simulink model "hx_sim"  (R2017b)
settings: Solver=ode23tb  StartTime=0.0  StopTime=tEndSimul  MaxStep=0.1  RelTol=5e-6
values from neighbouring files (symbols this model uses):
  dnDt_in = mass_flow_converter(0.020, 'kg/min', 'mol/sec', 'Ammonia')    [hx.m]
  dnDt_out_liq = mass_flow_converter(0.020, 'kg/min', 'mol/sec', 'Ammonia')    [hx.m]
  dnDt_out_vap = mass_flow_converter(0, 'kg/h', 'mol/sec', 'Ammonia')    [hx.m]
  fluid = nh3_v4    [hx.m]
  h_inner_liq = 1e2    (= 100)    [hx.m]
  h_inner_vap = 1e4    (= 10000)    [hx.m]
  h_outer = 200    [hx.m]
  Nhx_init = Vhx/10 * rho_nh3_Tamb    [hx.m]
  T_dnDt_in_C = 120    [hx.m]
  Tamb_C = 25    [hx.m]
  tEnd_dnDt_in = tStart_dnDt_in + 10 * c.min_to_sec    [hx.m]
  tEnd_dnDt_out_liq = tStart_dnDt_out_liq + 10 * c.min_to_sec    [hx.m]
  tEnd_dnDt_out_vap = tStart_dnDt_out_vap + 0 * c.min_to_sec    [hx.m]
  Thx_init = c.C_to_K(Tamb_C)    [hx.m]
  Tout1_C = (20+30)/2    (= 25)    [hx.m]
  tStart_dnDt_in = 10 * c.min_to_sec    [hx.m]
  tStart_dnDt_out_liq = tEnd_dnDt_in + 5 * c.min_to_sec    [hx.m]
  tStart_dnDt_out_vap = 0    [hx.m]
  Vhx = 0.5 * c.L_to_m3    [hx.m]
undefined symbols (not defined in the file or in its folder): h, P, T
libraries: thermochemical x19, simulink x4
settings Model: Creator=ferru  LastModifiedBy=fferrucc
settings SolverCC: AlgebraicLoopSolver=LineSearch

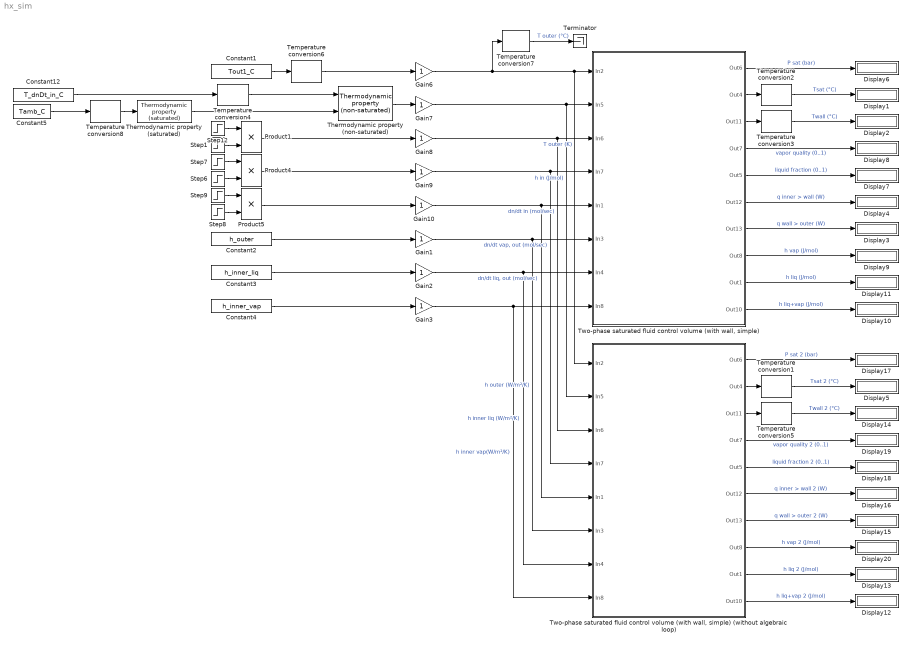
== system hx_sim ==
  Constant1 : Constant  Value=Tout1_C
  Constant12 : Constant  Value=T_dnDt_in_C
  Constant2 : Constant  Value=h_outer
  Constant3 : Constant  Value=h_inner_liq
  Constant4 : Constant  Value=h_inner_vap
  Constant5 : Constant  Value=Tamb_C
  Display{1..20} (20 alike) : Display
  Gain{1..3,6..10} (8 alike) : Gain
  Product1 : Product
  Product4 : Product
  Product5 : Product
  Step1 : Step  Time=tEnd_dnDt_in  Before=1  After=0  SampleTime=0
  Step12 : Step  Time=tStart_dnDt_in  After=dnDt_in  SampleTime=0
  Step6 : Step  Time=tEnd_dnDt_out_vap  Before=1  After=0  SampleTime=0
  Step7 : Step  Time=tStart_dnDt_out_vap  After=dnDt_out_vap  SampleTime=0
  Step8 : Step  Time=tEnd_dnDt_out_liq  Before=1  After=0  SampleTime=0
  Step9 : Step  Time=tStart_dnDt_out_liq  After=dnDt_out_liq  SampleTime=0
  Temperature conversion{1..3,5,7} (5 alike) : thermochemical/Conversions/Temperature conversion  sel=K --> °C
      settings: SourceProductName=@ Thermochemical
  Temperature conversion4 : thermochemical/Conversions/Temperature conversion  sel=°C --> K
      settings: SourceProductName=@ Thermochemical
  Temperature conversion6 : thermochemical/Conversions/Temperature conversion  sel=°C --> K
      settings: SourceProductName=@ Thermochemical
  Temperature conversion8 : thermochemical/Conversions/Temperature conversion  sel=°C --> K
      settings: SourceProductName=@ Thermochemical
  Terminator : Terminator
  Thermodynamic property (non-saturated) : thermochemical/Thermodynamic fluid properties/Thermodynamic  property (non-saturated)  sel=h(T,P)  fluid=fluid  reciprocVar=-1  lookup2D_BreakPoint1=fluid.no_sat.T_P_indep.var_indep.T  lookup2D_BreakPoint2=fluid.no_sat.T_P_indep.var_indep.P  lookup2D_Data=fluid.no_sat.T_P_indep.var_dep.h_molar
      settings: SourceProductName=@ Thermochemical
  Thermodynamic property (saturated) : thermochemical/Thermodynamic fluid properties/Thermodynamic  property (saturated)  sel=P(T) (bar)  fluid=fluid  lookup1D_BreakPoint1=fluid.sat.T  lookup1D_Data=fluid.sat.Psat
      settings: SourceProductName=@ Thermochemical
  "Two-phase saturated fluid control volume (with wall, simple)" : Subsystem  AncestorBlock=|
      | thermochemical/Control volumes/Two-phase saturated fluid
      | control volume (with wall, simple)
  "Two-phase saturated fluid control volume (with wall, simple) (without algebraic loop)" : Subsystem  AncestorBlock=|
      | thermochemical/Control volumes/Two-phase saturated fluid
      | control volume (with wall, simple)
      | (without algebraic loop)
  wires:
  Step12/1 -> Product1/1
  Step1/1 -> Product1/2
  Constant12/1 -> Temperature conversion4/1
  Temperature conversion4/1 -> Thermodynamic property (non-saturated)/1
  Temperature conversion2/1 -> Display1/1  "Tsat (°C)"
  "Two-phase saturated fluid control volume (with wall, simple)"/2(Out4) -> Temperature conversion2/1
  Gain6/1 -> Temperature conversion7/1, "Two-phase saturated fluid control volume (with wall, simple) (without algebraic loop)"/1(In2), "Two-phase saturated fluid control volume (with wall, simple)"/1(In2)  "T outer (K)"
  Gain7/1 -> "Two-phase saturated fluid control volume (with wall, simple) (without algebraic loop)"/2(In5), "Two-phase saturated fluid control volume (with wall, simple)"/2(In5)  "h in (J/mol)"
  Gain8/1 -> "Two-phase saturated fluid control volume (with wall, simple) (without algebraic loop)"/3(In6), "Two-phase saturated fluid control volume (with wall, simple)"/3(In6)  "dn/dt in (mol/sec)"
  Gain9/1 -> "Two-phase saturated fluid control volume (with wall, simple) (without algebraic loop)"/4(In7), "Two-phase saturated fluid control volume (with wall, simple)"/4(In7)  "dn/dt vap, out (mol/sec)"
  Gain10/1 -> "Two-phase saturated fluid control volume (with wall, simple) (without algebraic loop)"/5(In1), "Two-phase saturated fluid control volume (with wall, simple)"/5(In1)  "dn/dt liq, out (mol/sec)"
  "Two-phase saturated fluid control volume (with wall, simple)"/1(Out6) -> Display6/1  "P sat (bar)"
  "Two-phase saturated fluid control volume (with wall, simple)"/5(Out5) -> Display7/1  "liquid fraction (0..1)"
  "Two-phase saturated fluid control volume (with wall, simple)"/4(Out7) -> Display8/1  "vapor quality (0..1)"
  "Two-phase saturated fluid control volume (with wall, simple)"/8(Out8) -> Display9/1  "h vap (J/mol)"
  "Two-phase saturated fluid control volume (with wall, simple)"/10(Out10) -> Display10/1  "h liq+vap (J/mol)"
  "Two-phase saturated fluid control volume (with wall, simple)"/9(Out1) -> Display11/1  "h liq (J/mol)"
  Constant1/1 -> Temperature conversion6/1
  Thermodynamic property (non-saturated)/1 -> Gain7/1
  Product1/1 -> Gain8/1
  Product4/1 -> Gain9/1
  Step6/1 -> Product4/2
  Step7/1 -> Product4/1
  Step9/1 -> Product5/1
  Step8/1 -> Product5/2
  Product5/1 -> Gain10/1
  "Two-phase saturated fluid control volume (with wall, simple)"/3(Out11) -> Temperature conversion3/1
  Temperature conversion3/1 -> Display2/1  "Twall (°C)"
  "Two-phase saturated fluid control volume (with wall, simple)"/7(Out13) -> Display3/1  "q wall > outer (W)"
  "Two-phase saturated fluid control volume (with wall, simple)"/6(Out12) -> Display4/1  "q inner > wall (W)"
  "Two-phase saturated fluid control volume (with wall, simple) (without algebraic loop)"/6(Out12) -> Display16/1  "q inner > wall 2 (W)"
  "Two-phase saturated fluid control volume (with wall, simple) (without algebraic loop)"/7(Out13) -> Display15/1  "q wall > outer 2 (W)"
  Temperature conversion5/1 -> Display14/1  "Twall 2 (°C)"
  "Two-phase saturated fluid control volume (with wall, simple) (without algebraic loop)"/3(Out11) -> Temperature conversion5/1
  "Two-phase saturated fluid control volume (with wall, simple) (without algebraic loop)"/9(Out1) -> Display13/1  "h liq 2 (J/mol)"
  "Two-phase saturated fluid control volume (with wall, simple) (without algebraic loop)"/10(Out10) -> Display12/1  "h liq+vap 2 (J/mol)"
  "Two-phase saturated fluid control volume (with wall, simple) (without algebraic loop)"/8(Out8) -> Display20/1  "h vap 2 (J/mol)"
  "Two-phase saturated fluid control volume (with wall, simple) (without algebraic loop)"/4(Out7) -> Display19/1  "vapor quality 2 (0..1)"
  "Two-phase saturated fluid control volume (with wall, simple) (without algebraic loop)"/5(Out5) -> Display18/1  "liquid fraction 2 (0..1)"
  "Two-phase saturated fluid control volume (with wall, simple) (without algebraic loop)"/1(Out6) -> Display17/1  "P sat 2 (bar)"
  "Two-phase saturated fluid control volume (with wall, simple) (without algebraic loop)"/2(Out4) -> Temperature conversion1/1
  Temperature conversion1/1 -> Display5/1  "Tsat 2 (°C)"
  Temperature conversion6/1 -> Gain6/1
  Temperature conversion7/1 -> Terminator/1  "T outer (°C)"
  Gain3/1 -> "Two-phase saturated fluid control volume (with wall, simple) (without algebraic loop)"/8(In8), "Two-phase saturated fluid control volume (with wall, simple)"/8(In8)  "h inner vap(W/m²/K)"
  Gain1/1 -> "Two-phase saturated fluid control volume (with wall, simple)"/6(In3), "Two-phase saturated fluid control volume (with wall, simple) (without algebraic loop)"/6(In3)  "h outer (W/m²/K)"
  Gain2/1 -> "Two-phase saturated fluid control volume (with wall, simple) (without algebraic loop)"/7(In4), "Two-phase saturated fluid control volume (with wall, simple)"/7(In4)  "h inner liq (W/m²/K)"
  Constant2/1 -> Gain1/1
  Constant3/1 -> Gain2/1
  Constant4/1 -> Gain3/1
  Constant5/1 -> Temperature conversion8/1
  Temperature conversion8/1 -> Thermodynamic property (saturated)/1
  Thermodynamic property (saturated)/1 -> Thermodynamic property (non-saturated)/2

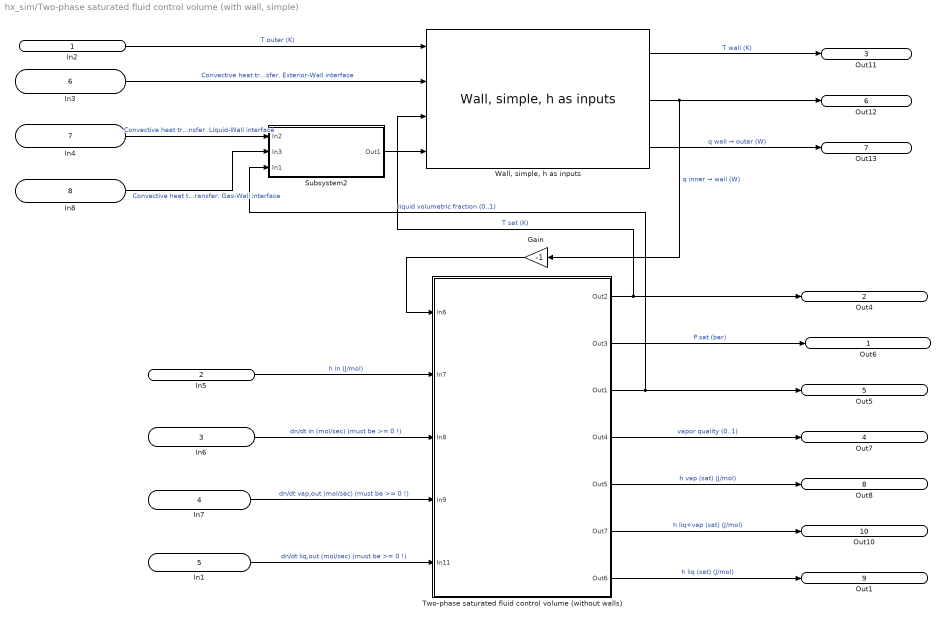
== system hx_sim/Two-phase saturated fluid control volume (with wall, simple) ==
  In2 : Inport
  In5 : Inport  Port=2
  In6 : Inport  Port=3
  In7 : Inport  Port=4
  In1 : Inport  Port=5
  In3 : Inport  Port=6
  In4 : Inport  Port=7
  In8 : Inport  Port=8
  Gain : Gain  Gain=-1
  Subsystem2 : Subsystem
  Two-phase saturated fluid control volume (without walls) : Subsystem  AncestorBlock=|  mask(volume_control_saturated){N_init=Nhx_init, T_init=Thx_init, fluid=fluid, V=Vhx}
      | thermochemical/Control volumes/Two-phase saturated fluid
      | control volume (without walls)
      mask prompts: N_init "Initial number of mols inside the control volume (mol)"; T_init "Fluid initial temperature (K)"; fluid "Fluid (structure data type)"; V "Volume (m3)"
      mask help:
      | This block models a volume control that contains a fluid always in its saturation state.
      |
      | The model can work as a condenser or as an evaporator:
      | • Condenser: connect the output 'h liq (J/mol)' to the input 'h out (sat) (J/mol)'
      | • Evaporator: connect the output 'h vap (J/mol)' to the input 'h out (sat) (J/mol)'
      |
      | The ratio between the two phases is given by two outputs:
      | 1) volumetric liquid fraction: liquid volume/total volume (0..1)
      | 2) vapor quality (e.g. zero: 100% liquid, one: 100% vapor).
      |
      | Note 2: the model is not prepared to work in the non-saturation state of the fluid (e.g. superheated gas or supercooled liquid). This means that both the liquid fraction and the vapor quality are strictly constrained in the (0..1) open range. The simulation will stop if these constrains are violated.
      mask DialogControl Container3 Prompt: Initial state
      mask DialogControl Container4 Prompt: Other parameters
  "Wall, simple, h as inputs" : thermochemical/Walls/Wall, simple, h as inputs  material=Stainless steel AISI316  cp=490.8  rho=8023  s=Shx_m2  e_mm=thickness_hx_mm  mass=2.2529  Twall_init=Thx_init
      settings: SourceProductName=@ Thermochemical
  Out6 : Outport
  Out4 : Outport  Port=2
  Out11 : Outport  Port=3
  Out7 : Outport  Port=4
  Out5 : Outport  Port=5
  Out12 : Outport  Port=6
  Out13 : Outport  Port=7
  Out8 : Outport  Port=8
  Out1 : Outport  Port=9
  Out10 : Outport  Port=10
  wires:
  Subsystem2/1(Out1) -> "Wall, simple, h as inputs"/4
  "Wall, simple, h as inputs"/2 -> Gain/1, Out12/1  "q inner → wall (W)"
  "Wall, simple, h as inputs"/1 -> Out11/1  "T wall (K)"
  In3/1 -> "Wall, simple, h as inputs"/2  "Convective heat transfer. Exterior-Wall interface"
  In4/1 -> Subsystem2/1(In2)  "Convective heat transfer. Liquid-Wall interface"
  Two-phase saturated fluid control volume (without walls)/7(Out6) -> Out1/1  "h liq (sat) (J/mol)"
  Two-phase saturated fluid control volume (without walls)/1(Out2) -> "Wall, simple, h as inputs"/3, Out4/1  "T sat (K)"
  Two-phase saturated fluid control volume (without walls)/2(Out3) -> Out6/1  "P sat (bar)"
  Two-phase saturated fluid control volume (without walls)/6(Out7) -> Out10/1  "h liq+vap (sat) (J/mol)"
  In7/1 -> Two-phase saturated fluid control volume (without walls)/4(In9)  "dn/dt vap,out (mol/sec) (must be >= 0 !)"
  Two-phase saturated fluid control volume (without walls)/5(Out5) -> Out8/1  "h vap (sat) (J/mol)"
  Two-phase saturated fluid control volume (without walls)/4(Out4) -> Out7/1  "vapor quality (0..1)"
  Two-phase saturated fluid control volume (without walls)/3(Out1) -> Subsystem2/3(In1), Out5/1  "liquid volumetric fraction (0..1)"
  In5/1 -> Two-phase saturated fluid control volume (without walls)/2(In7)  "h in (J/mol)"
  In6/1 -> Two-phase saturated fluid control volume (without walls)/3(In8)  "dn/dt in (mol/sec) (must be >= 0 !)"
  In8/1 -> Subsystem2/2(In3)  "Convective heat transfer. Gas-Wall interface"
  "Wall, simple, h as inputs"/3 -> Out13/1  "q wall → outer (W)"
  In2/1 -> "Wall, simple, h as inputs"/1  "T outer (K)"
  Gain/1 -> Two-phase saturated fluid control volume (without walls)/1(In6)
  In1/1 -> Two-phase saturated fluid control volume (without walls)/5(In11)  "dn/dt liq,out (mol/sec) (must be >= 0 !)"

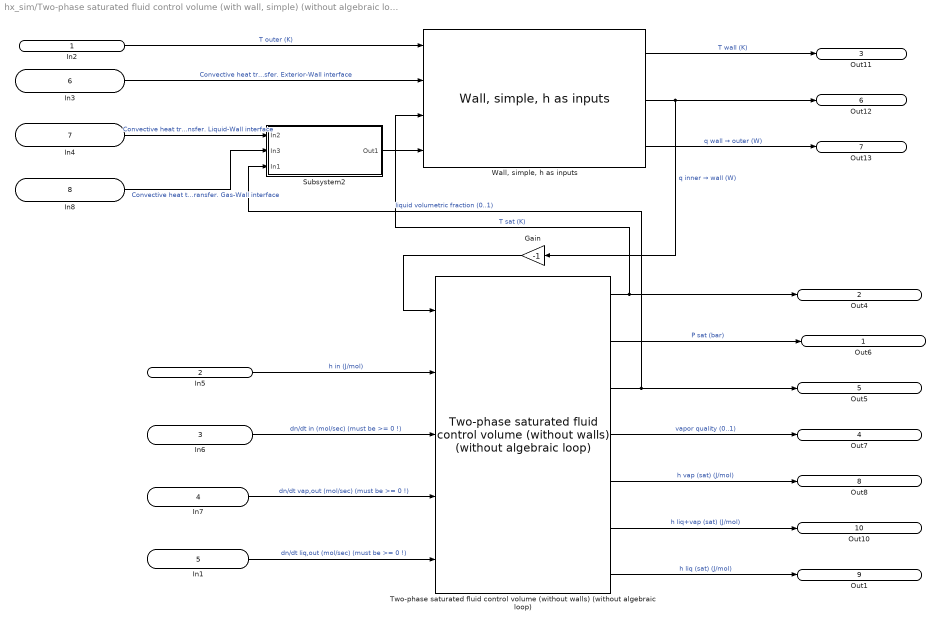
== system hx_sim/Two-phase saturated fluid control volume (with wall, simple) (without algebraic loop) ==
  In2 : Inport
  In5 : Inport  Port=2
  In6 : Inport  Port=3
  In7 : Inport  Port=4
  In1 : Inport  Port=5
  In3 : Inport  Port=6
  In4 : Inport  Port=7
  In8 : Inport  Port=8
  Gain : Gain  Gain=-1
  Subsystem2 : Subsystem
  Two-phase saturated fluid control volume (without walls) (without algebraic loop) : thermochemical/Control volumes/Two-phase saturated fluid control volume (without walls) (without algebraic loop)  N_init=Nhx_init  T_init=Thx_init  fluid=fluid  V=Vhx
      settings: SourceProductName=@ Thermochemical
  "Wall, simple, h as inputs" : thermochemical/Walls/Wall, simple, h as inputs  material=Stainless steel AISI316  cp=490.8  rho=8023  s=Shx_m2  e_mm=thickness_hx_mm  mass=2.2529  Twall_init=Thx_init
      settings: SourceProductName=@ Thermochemical
  Out6 : Outport
  Out4 : Outport  Port=2
  Out11 : Outport  Port=3
  Out7 : Outport  Port=4
  Out5 : Outport  Port=5
  Out12 : Outport  Port=6
  Out13 : Outport  Port=7
  Out8 : Outport  Port=8
  Out1 : Outport  Port=9
  Out10 : Outport  Port=10
  wires:
  In1/1 -> Two-phase saturated fluid control volume (without walls) (without algebraic loop)/5  "dn/dt liq,out (mol/sec) (must be >= 0 !)"
  Gain/1 -> Two-phase saturated fluid control volume (without walls) (without algebraic loop)/1
  In2/1 -> "Wall, simple, h as inputs"/1  "T outer (K)"
  "Wall, simple, h as inputs"/3 -> Out13/1  "q wall → outer (W)"
  In6/1 -> Two-phase saturated fluid control volume (without walls) (without algebraic loop)/3  "dn/dt in (mol/sec) (must be >= 0 !)"
  In5/1 -> Two-phase saturated fluid control volume (without walls) (without algebraic loop)/2  "h in (J/mol)"
  Two-phase saturated fluid control volume (without walls) (without algebraic loop)/3 -> Out5/1, Subsystem2/3(In1)  "liquid volumetric fraction (0..1)"
  Two-phase saturated fluid control volume (without walls) (without algebraic loop)/4 -> Out7/1  "vapor quality (0..1)"
  Two-phase saturated fluid control volume (without walls) (without algebraic loop)/5 -> Out8/1  "h vap (sat) (J/mol)"
  In7/1 -> Two-phase saturated fluid control volume (without walls) (without algebraic loop)/4  "dn/dt vap,out (mol/sec) (must be >= 0 !)"
  Two-phase saturated fluid control volume (without walls) (without algebraic loop)/6 -> Out10/1  "h liq+vap (sat) (J/mol)"
  Two-phase saturated fluid control volume (without walls) (without algebraic loop)/2 -> Out6/1  "P sat (bar)"
  Two-phase saturated fluid control volume (without walls) (without algebraic loop)/1 -> Out4/1, "Wall, simple, h as inputs"/3  "T sat (K)"
  Two-phase saturated fluid control volume (without walls) (without algebraic loop)/7 -> Out1/1  "h liq (sat) (J/mol)"
  "Wall, simple, h as inputs"/1 -> Out11/1  "T wall (K)"
  "Wall, simple, h as inputs"/2 -> Out12/1, Gain/1  "q inner → wall (W)"
  Subsystem2/1(Out1) -> "Wall, simple, h as inputs"/4
  In4/1 -> Subsystem2/1(In2)  "Convective heat transfer. Liquid-Wall interface"
  In3/1 -> "Wall, simple, h as inputs"/2  "Convective heat transfer. Exterior-Wall interface"
  In8/1 -> Subsystem2/2(In3)  "Convective heat transfer. Gas-Wall interface"

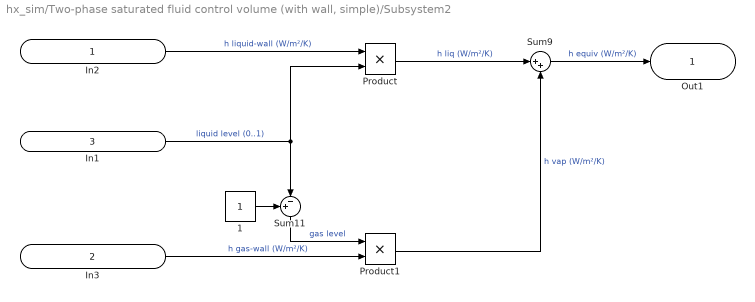
== system hx_sim/Two-phase saturated fluid control volume (with wall, simple)/Subsystem2 ==
  In2 : Inport
  In3 : Inport  Port=2
  In1 : Inport  Port=3
  1 : Constant
  Product : Product
  Product1 : Product
  Sum11 : Sum  Inputs=+-|
  Sum9 : Sum  Inputs=|++
  Out1 : Outport
  wires:
  Sum9/1 -> Out1/1  "h equiv (W/m²/K)"
  In1/1 -> Product/2, Sum11/2  "liquid level (0..1)"
  In3/1 -> Product1/2  "h gas-wall (W/m²/K)"
  In2/1 -> Product/1  "h liquid-wall (W/m²/K)"
  Sum11/1 -> Product1/1  "gas level"
  1/1 -> Sum11/1
  Product1/1 -> Sum9/2  "h vap (W/m²/K)"
  Product/1 -> Sum9/1  "h liq (W/m²/K)"

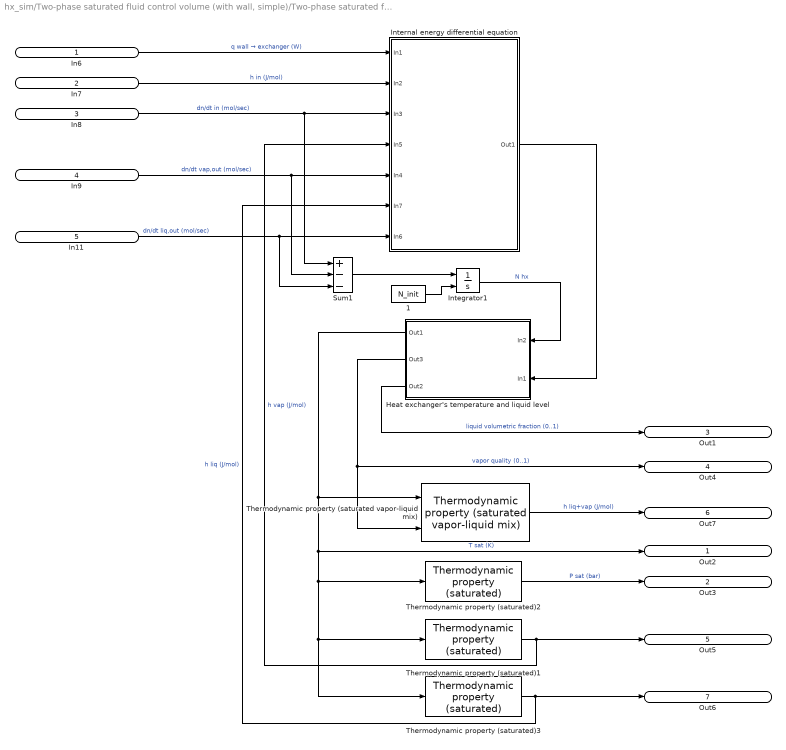
== system hx_sim/Two-phase saturated fluid control volume (with wall, simple)/Two-phase saturated fluid control volume (without walls) ==
  In6 : Inport
  In7 : Inport  Port=2
  In8 : Inport  Port=3
  In9 : Inport  Port=4
  In11 : Inport  Port=5
  1 : Constant  Value=N_init
  Heat exchanger's temperature and liquid level : Subsystem
  Integrator1 : Integrator  InitialConditionSource=external  InitialCondition=N_init
  Internal energy differential equation : Subsystem
  Sum1 : Sum  Inputs=+--
  Thermodynamic property (saturated)1 : thermochemical/Thermodynamic fluid properties/Thermodynamic  property (saturated)  sel=h(T) vap. (J/mol)  fluid=fluid  lookup1D_BreakPoint1=fluid.sat.T  lookup1D_Data=fluid.sat.vap.h_molar
      settings: SourceProductName=@ Thermochemical
  Thermodynamic property (saturated)2 : thermochemical/Thermodynamic fluid properties/Thermodynamic  property (saturated)  sel=P(T) (bar)  fluid=fluid  lookup1D_BreakPoint1=fluid.sat.T  lookup1D_Data=fluid.sat.Psat
      settings: SourceProductName=@ Thermochemical
  Thermodynamic property (saturated)3 : thermochemical/Thermodynamic fluid properties/Thermodynamic  property (saturated)  sel=h(T) liq. (J/mol)  fluid=fluid  lookup1D_BreakPoint1=fluid.sat.T  lookup1D_Data=fluid.sat.liq.h_molar
      settings: SourceProductName=@ Thermochemical
  Thermodynamic property (saturated vapor-liquid mix) : thermochemical/Thermodynamic fluid properties/Thermodynamic property  (saturated vapor-liquid mix)  sel=h(T) (J/mol)  fluid=fluid  lookup1D_BreakPoint=0  lookup1D_Data1=fluid.sat.liq.h_molar  lookup1D_Data2=fluid.sat.vap.h_molar
      settings: SourceProductName=@ Thermochemical
  Out2 : Outport
  Out3 : Outport  Port=2
  Out1 : Outport  Port=3
  Out4 : Outport  Port=4
  Out5 : Outport  Port=5
  Out7 : Outport  Port=6
  Out6 : Outport  Port=7
  wires:
  1/1 -> Integrator1/2
  In7/1 -> Internal energy differential equation/2(In2)  "h in (J/mol)"
  In11/1 -> Internal energy differential equation/7(In6), Sum1/3  "dn/dt liq,out (mol/sec)"
  In8/1 -> Internal energy differential equation/3(In3), Sum1/1  "dn/dt in (mol/sec)"
  In6/1 -> Internal energy differential equation/1(In1)  "q wall → exchanger (W)"
  In9/1 -> Internal energy differential equation/5(In4), Sum1/2  "dn/dt vap,out (mol/sec)"
  Thermodynamic property (saturated)3/1 -> Internal energy differential equation/6(In7), Out6/1  "h liq (J/mol)"
  Thermodynamic property (saturated vapor-liquid mix)/1 -> Out7/1  "h liq+vap (J/mol)"
  Thermodynamic property (saturated)1/1 -> Out5/1, Internal energy differential equation/4(In5)  "h vap (J/mol)"
  Internal energy differential equation/1(Out1) -> Heat exchanger's temperature and liquid level/2(In1)
  Integrator1/1 -> Heat exchanger's temperature and liquid level/1(In2)  "N hx"
  Heat exchanger's temperature and liquid level/2(Out3) -> Out4/1, Thermodynamic property (saturated vapor-liquid mix)/2  "vapor quality (0..1)"
  Thermodynamic property (saturated)2/1 -> Out3/1  "P sat (bar)"
  Heat exchanger's temperature and liquid level/1(Out1) -> Thermodynamic property (saturated vapor-liquid mix)/1, Out2/1, Thermodynamic property (saturated)2/1, Thermodynamic property (saturated)1/1, Thermodynamic property (saturated)3/1  "T sat (K)"
  Heat exchanger's temperature and liquid level/3(Out2) -> Out1/1  "liquid volumetric fraction (0..1)"
  Sum1/1 -> Integrator1/1

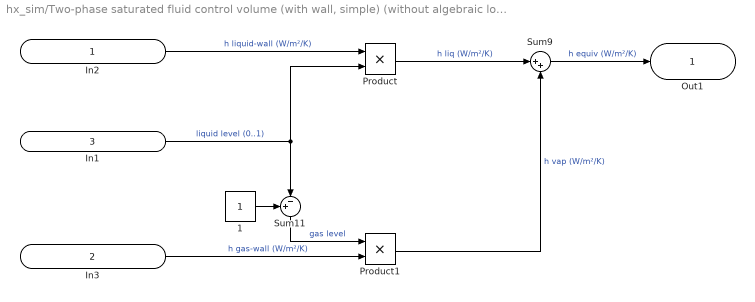
== system hx_sim/Two-phase saturated fluid control volume (with wall, simple) (without algebraic loop)/Subsystem2 ==
  In2 : Inport
  In3 : Inport  Port=2
  In1 : Inport  Port=3
  1 : Constant
  Product : Product
  Product1 : Product
  Sum11 : Sum  Inputs=+-|
  Sum9 : Sum  Inputs=|++
  Out1 : Outport
  wires:
  Product/1 -> Sum9/1  "h liq (W/m²/K)"
  Product1/1 -> Sum9/2  "h vap (W/m²/K)"
  1/1 -> Sum11/1
  Sum11/1 -> Product1/1  "gas level"
  In2/1 -> Product/1  "h liquid-wall (W/m²/K)"
  In3/1 -> Product1/2  "h gas-wall (W/m²/K)"
  In1/1 -> Sum11/2, Product/2  "liquid level (0..1)"
  Sum9/1 -> Out1/1  "h equiv (W/m²/K)"

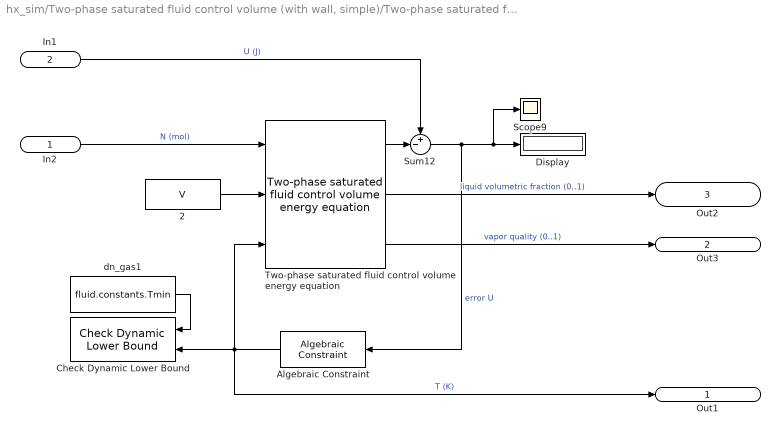
== system hx_sim/Two-phase saturated fluid control volume (with wall, simple)/Two-phase saturated fluid control volume (without walls)/Heat exchanger's temperature and liquid level ==
  In2 : Inport
  In1 : Inport  Port=2
  2 : Constant  Value=V
  Algebraic Constraint : AlgebraicConstraint  InitialGuess=T_init
  Check Dynamic Lower Bound : simulink/Model Verification/Check Dynamic  Lower Bound  Description=min < u  Enabled=on  stopWhenAssertionFail=on  export=off  icon=graphic
      settings: SourceProductName=Simulink  SourceProductBaseCode=SL
  Display : Display
  Scope9 : Scope
  Sum12 : Sum  Inputs=+-|
  Two-phase saturated fluid control volume energy equation : thermochemical/Control volumes/Two-phase saturated fluid control volume energy equation  fluid=fluid
      settings: SourceProductName=@ Thermochemical
  dn_gas1 : Constant  Value=fluid.constants.Tmin
  Out1 : Outport
  Out3 : Outport  Port=2
  Out2 : Outport  Port=3
  wires:
  2/1 -> Two-phase saturated fluid control volume energy equation/2
  Two-phase saturated fluid control volume energy equation/3 -> Out3/1  "vapor quality (0..1)"
  Two-phase saturated fluid control volume energy equation/1 -> Sum12/2
  Sum12/1 -> Algebraic Constraint/1, Display/1, Scope9/1  "error U"
  In1/1 -> Sum12/1  "U (J)"
  In2/1 -> Two-phase saturated fluid control volume energy equation/1  "N (mol)"
  dn_gas1/1 -> Check Dynamic Lower Bound/1
  Algebraic Constraint/1 -> Out1/1, Check Dynamic Lower Bound/2, Two-phase saturated fluid control volume energy equation/3  "T (K)"
  Two-phase saturated fluid control volume energy equation/2 -> Out2/1  "liquid volumetric fraction (0..1)"

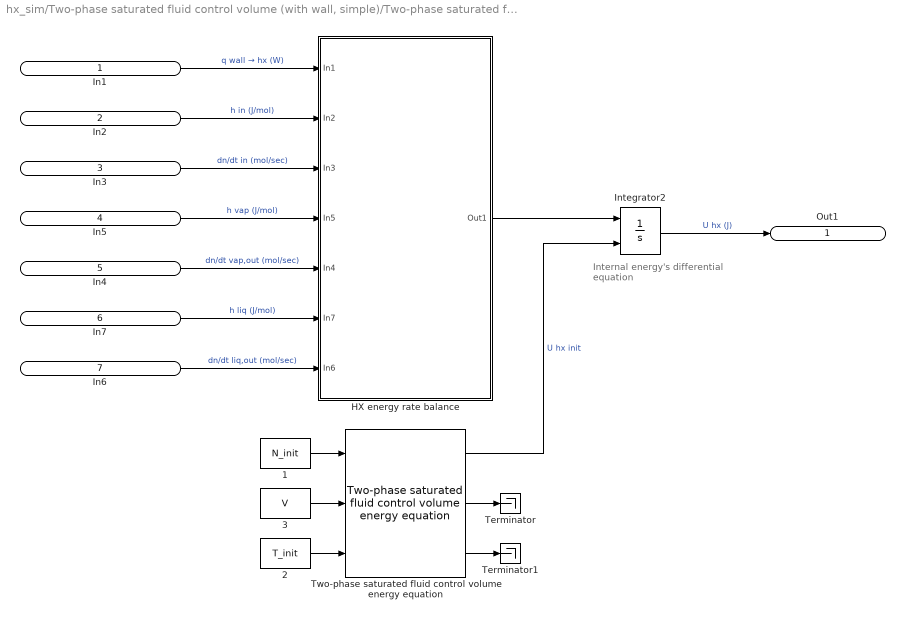
== system hx_sim/Two-phase saturated fluid control volume (with wall, simple)/Two-phase saturated fluid control volume (without walls)/Internal energy differential equation ==
  note: Internal energy's
      | differential equation
  In1 : Inport
  In2 : Inport  Port=2
  In3 : Inport  Port=3
  In5 : Inport  Port=4
  In4 : Inport  Port=5
  In7 : Inport  Port=6
  In6 : Inport  Port=7
  1 : Constant  Value=N_init
  2 : Constant  Value=T_init
  3 : Constant  Value=V
  HX energy rate balance : Subsystem
  Integrator2 : Integrator  InitialConditionSource=external
  Terminator : Terminator
  Terminator1 : Terminator
  Two-phase saturated fluid control volume energy equation : thermochemical/Control volumes/Two-phase saturated fluid control volume energy equation  fluid=fluid
      settings: SourceProductName=@ Thermochemical
  Out1 : Outport
  wires:
  HX energy rate balance/1(Out1) -> Integrator2/1
  In7/1 -> HX energy rate balance/6(In7)  "h liq (J/mol)"
  In5/1 -> HX energy rate balance/4(In5)  "h vap (J/mol)"
  In2/1 -> HX energy rate balance/2(In2)  "h in (J/mol)"
  In1/1 -> HX energy rate balance/1(In1)  "q wall → hx (W)"
  In6/1 -> HX energy rate balance/7(In6)  "dn/dt liq,out (mol/sec)"
  Two-phase saturated fluid control volume energy equation/3 -> Terminator1/1
  Two-phase saturated fluid control volume energy equation/2 -> Terminator/1
  3/1 -> Two-phase saturated fluid control volume energy equation/2
  Two-phase saturated fluid control volume energy equation/1 -> Integrator2/2  "U hx init"
  2/1 -> Two-phase saturated fluid control volume energy equation/3
  1/1 -> Two-phase saturated fluid control volume energy equation/1
  In3/1 -> HX energy rate balance/3(In3)  "dn/dt in (mol/sec)"
  In4/1 -> HX energy rate balance/5(In4)  "dn/dt vap,out (mol/sec)"
  Integrator2/1 -> Out1/1  "U hx (J)"

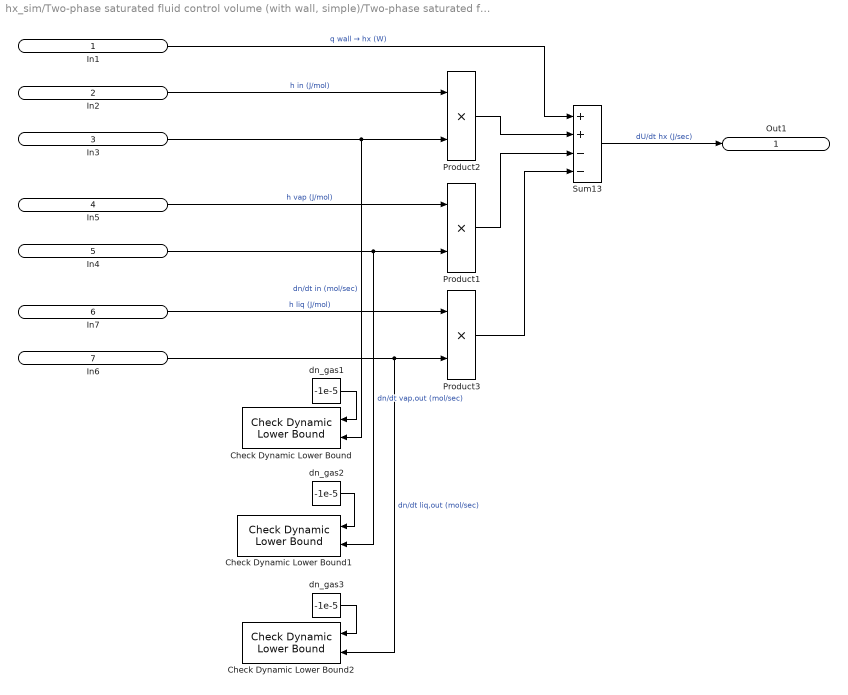
== system hx_sim/Two-phase saturated fluid control volume (with wall, simple)/Two-phase saturated fluid control volume (without walls)/Internal energy differential equation/HX energy rate balance ==
  In1 : Inport
  In2 : Inport  Port=2
  In3 : Inport  Port=3
  In5 : Inport  Port=4
  In4 : Inport  Port=5
  In7 : Inport  Port=6
  In6 : Inport  Port=7
  Check Dynamic Lower Bound : simulink/Model Verification/Check Dynamic  Lower Bound  Description=min < u  Enabled=on  stopWhenAssertionFail=on  export=off  icon=graphic
      settings: SourceProductName=Simulink  SourceProductBaseCode=SL
  Check Dynamic Lower Bound1 : simulink/Model Verification/Check Dynamic  Lower Bound  Description=min < u  Enabled=on  stopWhenAssertionFail=on  export=off  icon=graphic
      settings: SourceProductName=Simulink  SourceProductBaseCode=SL
  Check Dynamic Lower Bound2 : simulink/Model Verification/Check Dynamic  Lower Bound  Description=min < u  Enabled=on  stopWhenAssertionFail=on  export=off  icon=graphic
      settings: SourceProductName=Simulink  SourceProductBaseCode=SL
  Product1 : Product
  Product2 : Product
  Product3 : Product
  Sum13 : Sum  Inputs=++--
  dn_gas1 : Constant  Value=-1e-5
  dn_gas2 : Constant  Value=-1e-5
  dn_gas3 : Constant  Value=-1e-5
  Out1 : Outport
  wires:
  dn_gas1/1 -> Check Dynamic Lower Bound/1
  dn_gas3/1 -> Check Dynamic Lower Bound2/1
  dn_gas2/1 -> Check Dynamic Lower Bound1/1
  In6/1 -> Product3/2, Check Dynamic Lower Bound2/2  "dn/dt liq,out (mol/sec)"
  In5/1 -> Product1/1  "h vap (J/mol)"
  In1/1 -> Sum13/1  "q wall → hx (W)"
  In2/1 -> Product2/1  "h in (J/mol)"
  In7/1 -> Product3/1  "h liq (J/mol)"
  In3/1 -> Product2/2, Check Dynamic Lower Bound/2  "dn/dt in (mol/sec)"
  In4/1 -> Product1/2, Check Dynamic Lower Bound1/2  "dn/dt vap,out (mol/sec)"
  Product3/1 -> Sum13/4
  Product1/1 -> Sum13/3
  Product2/1 -> Sum13/2
  Sum13/1 -> Out1/1  "dU/dt hx (J/sec)"
